simulink model "USV_tracking"  (R2023b)
settings: Solver=FixedStepAuto  StartTime=0.0  StopTime=80  FixedStep=0.001  MaxStep=1e-3  RelTol=1e-5
InitFcn:
  | USV_tracking_init
StopFcn:
  | USV_tracking_stop
values from neighbouring files (symbols this model uses):
  d11 = 3.436    [USV_tracking_init.m]
  d22 = 12.99    [USV_tracking_init.m]
  d33 = 0.864    [USV_tracking_init.m]
  m11 = 1.412    [USV_tracking_init.m]
  m22 = 1.982    [USV_tracking_init.m]
  m33 = 0.354    [USV_tracking_init.m]
  th0 = 0    [USV_tracking_init.m]
  th1 = 2    [USV_tracking_init.m]    (also in USV_tracking_stop.m = simout1(:,4))
  vx0 = 0    [USV_tracking_init.m]
  vx1 = 0    [USV_tracking_init.m]    (also in USV_tracking_stop.m = simout1(:,5))
  vy0 = 0    [USV_tracking_init.m]
  vy1 = 0    [USV_tracking_init.m]    (also in USV_tracking_stop.m = simout1(:,6))
  w0 = 0    [USV_tracking_init.m]
  w1 = 0    [USV_tracking_init.m]    (also in USV_tracking_stop.m = simout1(:,7))
  x0 = 0    [USV_tracking_init.m]
  x1 = 5    [USV_tracking_init.m]    (also in USV_tracking_stop.m = simout1(:,2))
  y0 = 0    [USV_tracking_init.m]
  y1 = -3    [USV_tracking_init.m]    (also in USV_tracking_stop.m = simout1(:,3))
settings Model: SimulationMode=accelerator  PacingRate=4  Creator=bwang  LastModifiedBy=bwang-ccny
settings SolverCC: AlgebraicLoopSolver=LineSearch
settings DataIOCC: ReturnWorkspaceOutputs=off
settings DebuggingCC: UnconnectedInputMsg=warning  UnconnectedOutputMsg=warning  UnconnectedLineMsg=warning  ArithmeticOperatorsInVariantConditions=warning
settings HardwareCC: ProdBitPerLong=64  ProdHWDeviceType=Intel->x86-64 (Linux 64)
settings ModelReferenceCC: EnableRefExpFcnMdlSchedulingChecks=on
settings SFSimCC: SimUseLocalCustomCode=off  CustomCodeUndefinedFunction=UseInterfaceOnly
settings RTWCC: RTWUseLocalCustomCode=off  DLArmComputeVersion=19.05
settings CodeAppCC: MaxIdLength=95

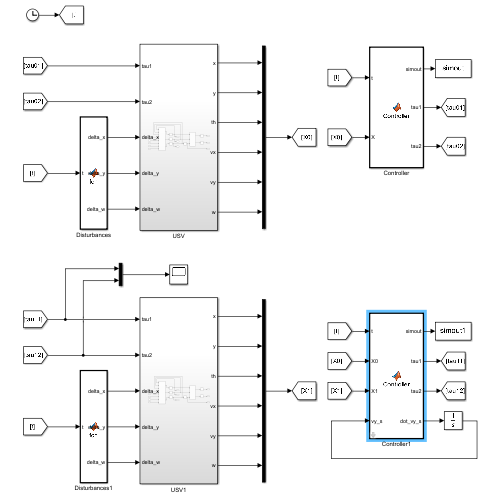
[thumbnail: Simulink's stored preview of the top-level diagram]
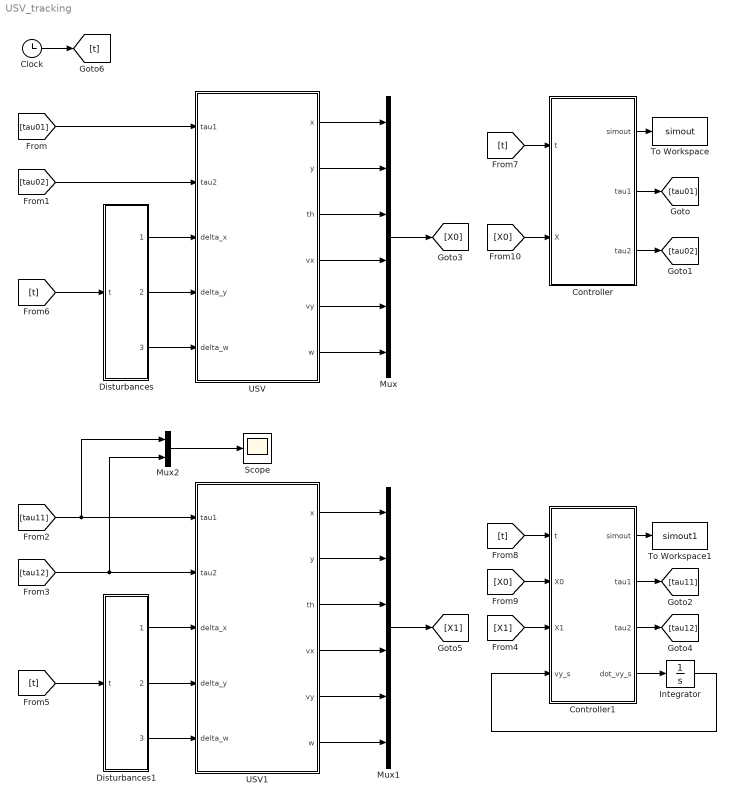
== system USV_tracking ==
  Clock : Clock
  Controller : MATLAB Function  TreatAsAtomicUnit=on
  Controller1 : MATLAB Function  TreatAsAtomicUnit=on  mask{m11=m11, m22=m22, m33=m33, d11=d11, d22=d22, d33=d33}
  Disturbances : MATLAB Function  TreatAsAtomicUnit=on
  Disturbances1 : MATLAB Function  TreatAsAtomicUnit=on
  Integrator : Integrator  InitialCondition=vy0
  Mux : Mux  Inputs=6
  Mux1 : Mux  Inputs=6
  Mux2 : Mux  Inputs=2
  Scope : Scope
  To Workspace : ToWorkspace  VariableName=simout  SampleTime=-1
      settings: Save2DSignal=2-D array (concatenate along first dimension)
  To Workspace1 : ToWorkspace  VariableName=simout1  SampleTime=-1
      settings: Save2DSignal=2-D array (concatenate along first dimension)
  USV : Subsystem
  USV1 : Subsystem
  wires:
  [t] -> Controller/1(t)
  [t] -> Disturbances/1(t)
  Disturbances/2(delta_y) -> USV/4(delta_y)
  Controller/2(tau1) -> [tau01]
  Controller/3(tau2) -> [tau02]
  Clock/1 -> [t]
  Disturbances/1(delta_x) -> USV/3(delta_x)
  Disturbances/3(delta_w) -> USV/5(delta_w)
  USV/5(vy) -> Mux/5
  USV/4(vx) -> Mux/4
  USV/3(th) -> Mux/3
  USV/1(x) -> Mux/1
  USV/2(y) -> Mux/2
  USV/6(w) -> Mux/6
  Mux/1 -> [X0]
  [X0] -> Controller/2(X)
  Controller/1(simout) -> To Workspace/1
  [tau01] -> USV/1(tau1)
  [tau02] -> USV/2(tau2)
  USV1/4(vx) -> Mux1/4
  Disturbances1/1(delta_x) -> USV1/3(delta_x)
  [t] -> Controller1/1(t)
  Disturbances1/2(delta_y) -> USV1/4(delta_y)
  [t] -> Disturbances1/1(t)
  USV1/3(th) -> Mux1/3
  [tau11] -> Mux2/1, USV1/1(tau1)
  [tau12] -> Mux2/2, USV1/2(tau2)
  USV1/1(x) -> Mux1/1
  USV1/5(vy) -> Mux1/5
  Disturbances1/3(delta_w) -> USV1/5(delta_w)
  Controller1/2(tau1) -> [tau11]
  Controller1/3(tau2) -> [tau12]
  USV1/2(y) -> Mux1/2
  USV1/6(w) -> Mux1/6
  Controller1/1(simout) -> To Workspace1/1
  Mux1/1 -> [X1]
  [X1] -> Controller1/3(X1)
  [X0] -> Controller1/2(X0)
  Controller1/4(dot_vy_s) -> Integrator/1
  Integrator/1 -> Controller1/4(vy_s)
  Mux2/1 -> Scope/1

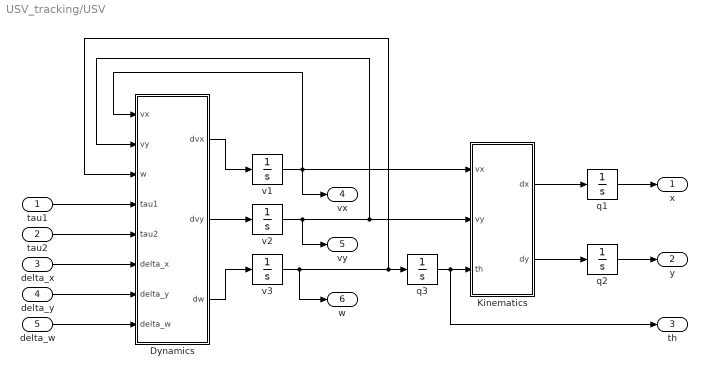
== system USV_tracking/USV ==
  tau1 : Inport
  tau2 : Inport  Port=2
  delta_x : Inport  Port=3
  delta_y : Inport  Port=4
  delta_w : Inport  Port=5
  Dynamics : MATLAB Function  TreatAsAtomicUnit=on  mask{m11=m11, m22=m22, m33=m33, d11=d11, d22=d22, d33=d33}
  Kinematics : MATLAB Function  TreatAsAtomicUnit=on
  q1 : Integrator  InitialCondition=x0
  q2 : Integrator  InitialCondition=y0
  q3 : Integrator  InitialCondition=th0
  v1 : Integrator  InitialCondition=vx0
  v2 : Integrator  InitialCondition=vy0
  v3 : Integrator  InitialCondition=w0
  x : Outport  VectorParamsAs1DForOutWhenUnconnected=off
  y : Outport  Port=2  VectorParamsAs1DForOutWhenUnconnected=off
  th : Outport  Port=3  VectorParamsAs1DForOutWhenUnconnected=off
  vx : Outport  Port=4  VectorParamsAs1DForOutWhenUnconnected=off
  vy : Outport  Port=5  VectorParamsAs1DForOutWhenUnconnected=off
  w : Outport  Port=6  VectorParamsAs1DForOutWhenUnconnected=off
  wires:
  Kinematics/2(dy) -> q2/1
  delta_w/1 -> Dynamics/8(delta_w)
  Dynamics/3(dw) -> v3/1
  v1/1 -> vx/1, Dynamics/1(vx), Kinematics/1(vx)
  q3/1 -> th/1, Kinematics/3(th)
  Kinematics/1(dx) -> q1/1
  v3/1 -> w/1, Dynamics/3(w), q3/1
  tau2/1 -> Dynamics/5(tau2)
  q2/1 -> y/1
  v2/1 -> vy/1, Kinematics/2(vy), Dynamics/2(vy)
  Dynamics/2(dvy) -> v2/1
  delta_y/1 -> Dynamics/7(delta_y)
  Dynamics/1(dvx) -> v1/1
  delta_x/1 -> Dynamics/6(delta_x)
  tau1/1 -> Dynamics/4(tau1)
  q1/1 -> x/1

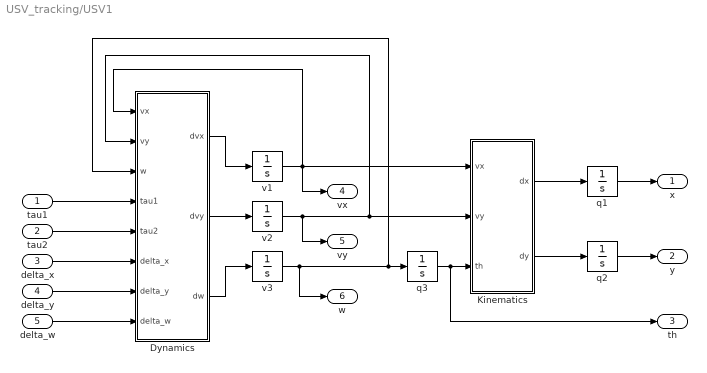
== system USV_tracking/USV1 ==
  tau1 : Inport
  tau2 : Inport  Port=2
  delta_x : Inport  Port=3
  delta_y : Inport  Port=4
  delta_w : Inport  Port=5
  Dynamics : MATLAB Function  TreatAsAtomicUnit=on  mask{m11=m11, m22=m22, m33=m33, d11=d11, d22=d22, d33=d33}
  Kinematics : MATLAB Function  TreatAsAtomicUnit=on
  q1 : Integrator  InitialCondition=x1
  q2 : Integrator  InitialCondition=y1
  q3 : Integrator  InitialCondition=th1
  v1 : Integrator  InitialCondition=vx1
  v2 : Integrator  InitialCondition=vy1
  v3 : Integrator  InitialCondition=w1
  x : Outport  VectorParamsAs1DForOutWhenUnconnected=off
  y : Outport  Port=2  VectorParamsAs1DForOutWhenUnconnected=off
  th : Outport  Port=3  VectorParamsAs1DForOutWhenUnconnected=off
  vx : Outport  Port=4  VectorParamsAs1DForOutWhenUnconnected=off
  vy : Outport  Port=5  VectorParamsAs1DForOutWhenUnconnected=off
  w : Outport  Port=6  VectorParamsAs1DForOutWhenUnconnected=off
  wires:
  Kinematics/2(dy) -> q2/1
  delta_w/1 -> Dynamics/8(delta_w)
  Dynamics/3(dw) -> v3/1
  v1/1 -> vx/1, Dynamics/1(vx), Kinematics/1(vx)
  q3/1 -> th/1, Kinematics/3(th)
  Kinematics/1(dx) -> q1/1
  v3/1 -> w/1, Dynamics/3(w), q3/1
  tau2/1 -> Dynamics/5(tau2)
  q2/1 -> y/1
  v2/1 -> vy/1, Kinematics/2(vy), Dynamics/2(vy)
  Dynamics/2(dvy) -> v2/1
  delta_y/1 -> Dynamics/7(delta_y)
  Dynamics/1(dvx) -> v1/1
  delta_x/1 -> Dynamics/6(delta_x)
  tau1/1 -> Dynamics/4(tau1)
  q1/1 -> x/1

== matlab function USV_tracking/Disturbances1 ==
  data: t input; delta_x output; delta_y output; delta_w output
function [delta_x, delta_y, delta_w] = fcn(t)

delta_x = 0;
delta_y = 0;
delta_w = 0;

== matlab function USV_tracking/USV1/Dynamics ==
  data: vx input; dvx output; vy input; w input; tau1 input; tau2 input; dvy output; dw output; delta_x input; delta_y input; delta_w input; m11 parameter; m22 parameter; m33 parameter; d11 parameter; d22 parameter; d33 parameter
function [dvx, dvy, dw] = fcn(vx, vy, w, tau1, tau2, delta_x, delta_y, delta_w, m11, m22, m33, d11, d22, d33)

%% USV: linear damping

fx = (m22/m11)*vy*w - (d11/m11)*vx;
fy = (-m11/m22)*vx*w - (d22/m22)*vy;
fw = ((m11 - m22)/m33)*vx*vy - (d33/m33)*w;


%% Plant
dvx = fx + delta_x + tau1/m11;
dvy = fy + delta_y;
dw = fw + delta_w + tau2/m33;

== matlab function USV_tracking/USV1/Kinematics ==
  data: vx input; dx output; vy input; th input; dy output
function [dx,dy] = fcn(vx, vy, th)

dx = vx*cos(th) - vy*sin(th);
dy = vx*sin(th) + vy*cos(th);

== matlab function USV_tracking/USV/Dynamics ==
  data: vx input; dvx output; vy input; w input; tau1 input; tau2 input; dvy output; dw output; delta_x input; delta_y input; delta_w input; m11 parameter; m22 parameter; m33 parameter; d11 parameter; d22 parameter; d33 parameter
function [dvx, dvy, dw] = fcn(vx, vy, w, tau1, tau2, delta_x, delta_y, delta_w, m11, m22, m33, d11, d22, d33)

%% USV: linear damping

fx = (m22/m11)*vy*w - (d11/m11)*vx;
fy = (-m11/m22)*vx*w - (d22/m22)*vy;
fw = ((m11 - m22)/m33)*vx*vy - (d33/m33)*w;


%% Plant
dvx = fx + delta_x + tau1/m11;
dvy = fy + delta_y;
dw = fw + delta_w + tau2/m33;

== matlab function USV_tracking/USV/Kinematics ==
  data: vx input; dx output; vy input; th input; dy output
function [dx,dy] = fcn(vx, vy, th)

dx = vx*cos(th) - vy*sin(th);
dy = vx*sin(th) + vy*cos(th);

== matlab function USV_tracking/Controller ==
  data: simout output; t input; X input size=[1,6]; tau1 output; tau2 output
function [simout, tau1,tau2] = Controller(t, X)

%% State variables
x = X(1);
y = X(2);
th = X(3);
vx = X(4);
vy = X(5);
w = X(6);

%% Control input

% Sine
tau1 = 2;
tau2 = 0.2*sin(0.2*t);

% % Circle
% tau1 = 2;
% tau2 = 0.5;

simout = [t, x, y, th, vx, vy, w, tau1, tau2];
end

== matlab function USV_tracking/Disturbances ==
  data: t input; delta_x output; delta_y output; delta_w output
function [delta_x, delta_y, delta_w] = fcn(t)

delta_x = 0;
delta_y = 0;
delta_w = 0;

== matlab function USV_tracking/Controller1 ==
  data: simout output size=[1 9]; t input; X0 input size=[1,6]; tau1 output size=1; tau2 output size=1; X1 input; vy_s input size=1; dot_vy_s output size=1; m11 parameter; m22 parameter; m33 parameter; d11 parameter; d22 parameter; d33 parameter
function [simout, tau1, tau2, dot_vy_s] = Controller(t, X0, X1, vy_s, m11, m22, m33, d11, d22, d33)


%% State variables
xd = X0(1);
yd = X0(2);
thd = X0(3);
vxd = X0(4);
vyd = X0(5);
wd = X0(6);

x = X1(1);
y = X1(2);
th = X1(3);
vx = X1(4);
vy = X1(5);
w = X1(6);

%% Parameters

%% Errors
ex = cos(th)*(x - xd) + sin(th)*(y - yd);
ey = -sin(th)*(x - xd) + cos(th)*(y - yd);
eth = th - thd;

dot_ex = w*ey + vx - vxd*cos(eth) - vyd*sin(eth);
dot_eth = w - wd;

kx = 0.2;
kth = 0.2;

vx_s = vxd - kx*(ex);
w_s = wd - kth*eth;

dot_vx_s = -kx*dot_ex;
dot_w_s = -kth*dot_eth;

%% Control input

kdx = 10;
kdw = 10;

tau1 = m11*dot_vx_s - m22*vy*w_s + d11*vx_s - kdx*(vx - vx_s);
tau2 = m33*dot_w_s + m22*vy*vx_s - m11*vx*vy_s + d33*w_s - kdw*(w - w_s);

dot_vy_s = -m11/m22*vx_s*w_s - d22/m22*vy_s;

simout = [t, x, y, th, vx, vy, w, tau1, tau2];
end

function y = sat(x,a)

if abs(x) >= a
    y = sign(x)*a;
else
    y = x;
end

end
